simulink model "sin3t"  (R2018b)
settings: Solver=VariableStepAuto  StartTime=0.0  StopTime=50  RelTol=1e-3
libraries: cstblocks x2
settings Model: Creator=Oguz  LastModifiedBy=Oguz

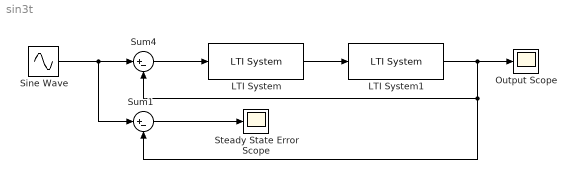
== system sin3t ==
  LTI System : cstblocks/LTI System  sys=P  IC=[]
  LTI System1 : cstblocks/LTI System  sys=C  IC=[]
  "Output Scope " : Scope
      settings: Description=Output Scope
  Sine Wave : Sin  Frequency=3  SampleTime=0
  Steady State Error Scope : Scope
  Sum1 : Sum  Inputs=|+-
  Sum4 : Sum  Inputs=|+-
  wires:
  LTI System/1 -> LTI System1/1
  LTI System1/1 -> "Output Scope "/1, Sum1/2, Sum4/2
  Sine Wave/1 -> Sum1/1, Sum4/1
  Sum4/1 -> LTI System/1
  Sum1/1 -> Steady State Error Scope/1
